simulink model "Ex3s"  (R2025a)
settings: Solver=VariableStepAuto  StartTime=0.0  StopTime=30  RelTol=1e-3
undefined symbols (not defined in the file): dend, numd

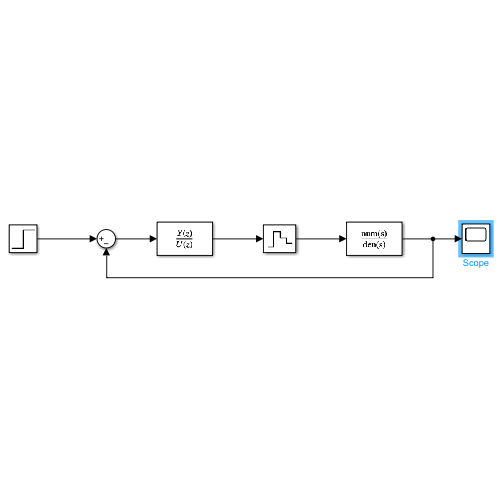
[thumbnail: Simulink's stored preview of the top-level diagram]
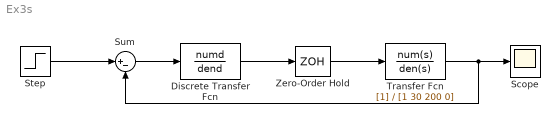
== system Ex3s ==
  Discrete Transfer Fcn : DiscreteTransferFcn  Numerator=numd  Denominator=dend
  Scope : Scope
      settings: ActiveDisplayYMinimum=-0.11454440585612445  ActiveDisplayYMaximum=1.0308996527051204
  Step : Step  SampleTime=0
  Sum : Sum  Inputs=|+-  SampleTime=0.1
  Transfer Fcn : TransferFcn  Denominator=[1 30 200 0]
  Zero-Order Hold : ZeroOrderHold  SampleTime=-1
  wires:
  Transfer Fcn/1 -> Sum/2, Scope/1
  Zero-Order Hold/1 -> Transfer Fcn/1
  Discrete Transfer Fcn/1 -> Zero-Order Hold/1
  Step/1 -> Sum/1
  Sum/1 -> Discrete Transfer Fcn/1
